simulink model "CRDI_CR"  (R2019a)
settings: Solver=VariableStepAuto  StartTime=0.0  StopTime=10.0  RelTol=1e-3
settings Model: Creator=user  LastModifiedBy=user

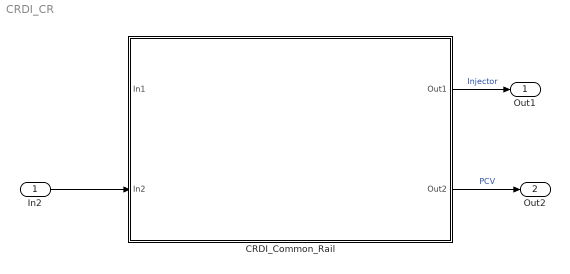
== system CRDI_CR ==
  In2 : Inport
  CRDI_Common_Rail : Subsystem
  Out1 : Outport
  Out2 : Outport  Port=2
  wires:
  In2/1 -> CRDI_Common_Rail/2(In2)
  CRDI_Common_Rail/1(Out1) -> Out1/1  "Injector"
  CRDI_Common_Rail/2(Out2) -> Out2/1  "PCV"

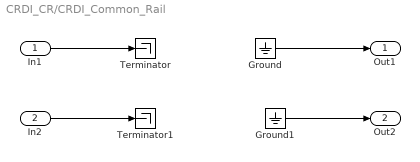
== system CRDI_CR/CRDI_Common_Rail ==
  In1 : Inport
  In2 : Inport  Port=2
  Ground : Ground
  Ground1 : Ground
  Terminator : Terminator
  Terminator1 : Terminator
  Out1 : Outport
  Out2 : Outport  Port=2
  wires:
  Ground/1 -> Out1/1
  Ground1/1 -> Out2/1
  In2/1 -> Terminator1/1
  In1/1 -> Terminator/1
